simulink model "Follow_Gap_Computation_2023a"  (R2023a)
settings: Solver=ode3  StartTime=0.0  StopTime=inf  FixedStep=0.05  RelTol=1e-3
libraries: robotlib x4
settings Model: Creator=pmodi  LastModifiedBy=gptp
settings OptimizationCC: EnhancedBackFolding=on  PassReuseOutputArgsAs=Individual arguments  ZeroExternalMemoryAtStartup=off  ZeroInternalMemoryAtStartup=off  MaxStackSize=64  OptimizeBlockOrder=speed  DifferentSizesBufferReuse=on  OptimizationCustomize=off  EfficientTunableParamExpr=on
settings DebuggingCC: ParameterTunabilityLossMsg=error
settings HardwareCC: ProdBitPerLong=64  ProdLargestAtomicInteger=LongLong  ProdLargestAtomicFloat=Double  ProdLongLongMode=on  ProdHWDeviceType=ARM Compatible->ARM 64-bit (LP64)
settings SFSimCC: MATLABDynamicMemAlloc=off
settings RTWCC: Description=Embedded Coder  SystemTargetFile=ert.tlc  HardwareBoard=Robot Operating System (ROS)  TLCOptions="-aInlineSetEventsForThisBaseRateFcn=TLC_FALSE -aSuppressMultiTaskScheduler=TLC_FALSE  -aRateBasedStepFcn=0"  GenCodeOnly=on  TemplateMakefile=ert_default_tmf  Toolchain=Catkin  TargetLang=C++
settings CodeAppCC: ForceParamTrailComments=on  IgnoreCustomStorageClasses=off  OperatorAnnotations=on  SimulinkDataObjDesc=on  SFDataObjDesc=on  InsertBlockDesc=on
settings ERTTargetCC: SupportVariableSizeSignals=on

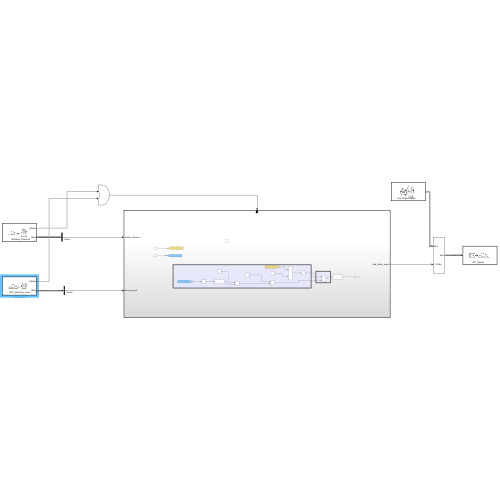
[thumbnail: Simulink's stored preview of the top-level diagram]
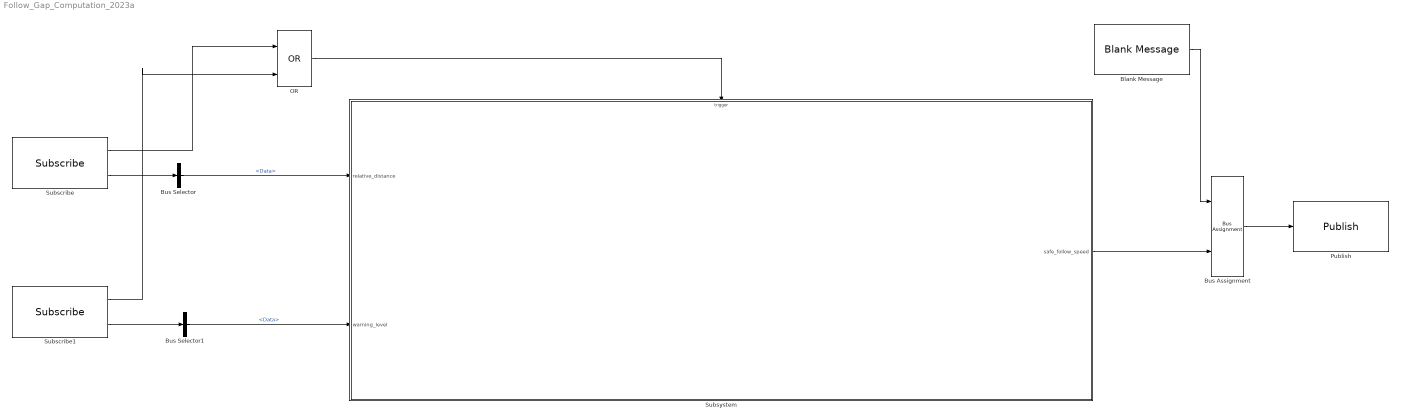
== system Follow_Gap_Computation_2023a ==
  Blank Message : robotlib/Blank Message  messageClass=Message  entityType=std_msgs/Float32  messageType=std_msgs/Float32  SampleTime=inf  legacyBusStruct=off
  Bus Assignment : BusAssignment  AssignedSignals=Data
  Bus Selector : BusSelector  OutputSignals=Data
  Bus Selector1 : BusSelector  OutputSignals=Data
  OR : Logic  Operator=OR  IconShape=distinctive  AllPortsSameDT=off  OutDataTypeStr=boolean
  Publish : robotlib/Publish  topicSource=Specify your own  topic=/SF_Speed  messageType=std_msgs/Float32  legacyBusStruct=off  messageQueueLength=1
  Subscribe : robotlib/Subscribe  topicSource=Specify your own  topic=/Relative_Distance  messageType=std_msgs/Float32  SampleTime=-1  legacyBusStruct=off  messageQueueLength=1
  Subscribe1 : robotlib/Subscribe  topicSource=Specify your own  topic=/V2V_Warning_Level  messageType=std_msgs/UInt8  SampleTime=-1  legacyBusStruct=off  messageQueueLength=1
  Subsystem : Subsystem
  wires:
  Subscribe/2 -> Bus Selector/1
  Bus Selector/1 -> Subsystem/1(relative_distance)  "<Data>"
  Bus Selector1/1 -> Subsystem/2(warning_level)  "<Data>"
  Subscribe1/2 -> Bus Selector1/1
  Blank Message/1 -> Bus Assignment/1
  Subsystem/1(safe_follow_speed) -> Bus Assignment/2
  Bus Assignment/1 -> Publish/1
  Subscribe/1 -> OR/1
  Subscribe1/1 -> OR/2
  OR/1 -> Subsystem/Trigger

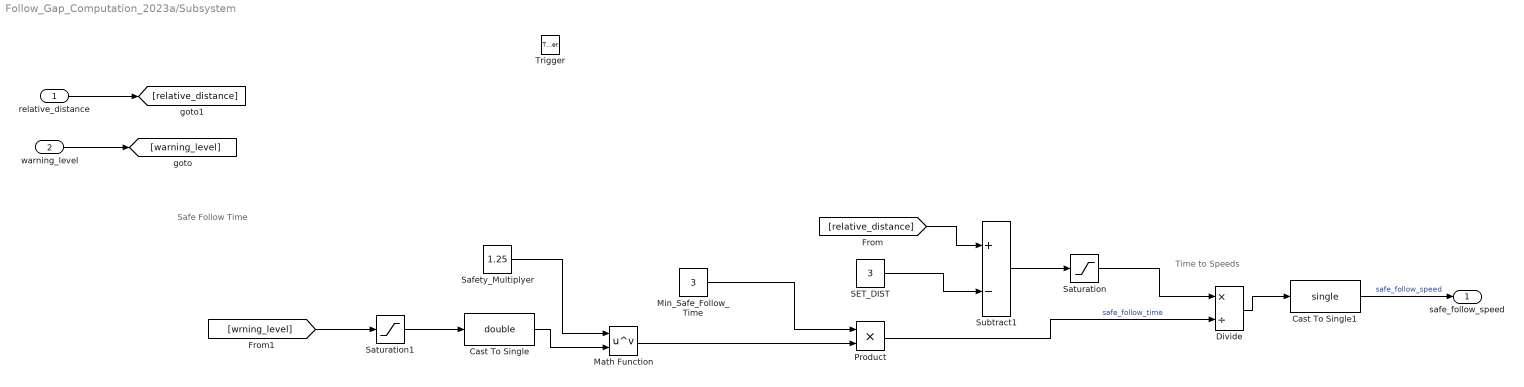
== system Follow_Gap_Computation_2023a/Subsystem ==
  note: Time to Speeds
  note: Safe Follow Time
  relative_distance : Inport
  warning_level : Inport  Port=2  OutDataTypeStr=uint8
  Trigger : TriggerPort  VariantControl=(inherit)  PortDimensions=1
  Cast To Single : DataTypeConversion  OutDataTypeStr=double  SaturateOnIntegerOverflow=off  RndMeth=Floor
  Cast To Single1 : DataTypeConversion  OutDataTypeStr=single  SaturateOnIntegerOverflow=off  RndMeth=Floor
  Divide : Product  Inputs=*/
  Math Function : Math  Operator=pow
  Min_Safe_Follow_Time : Constant  Value=3
  Product : Product
  SET_DIST : Constant  Value=3
  Safety_Multiplyer : Constant  Value=1.25
  Saturation : Saturate  UpperLimit=inf  LowerLimit=0
  Saturation1 : Saturate  UpperLimit=10  LowerLimit=0
  Subtract1 : Sum  Inputs=+-
  safe_follow_speed : Outport  OutDataTypeStr=single
  wires:
  Subtract1/1 -> Saturation/1
  Divide/1 -> Cast To Single1/1
  [relative_distance] -> Subtract1/1
  Math Function/1 -> Product/2
  Saturation/1 -> Divide/1
  relative_distance/1 -> [relative_distance]
  SET_DIST/1 -> Subtract1/2
  warning_level/1 -> [warning_level]
  Safety_Multiplyer/1 -> Math Function/1
  Min_Safe_Follow_Time/1 -> Product/1
  Cast To Single/1 -> Math Function/2
  [wrning_level] -> Saturation1/1
  Saturation1/1 -> Cast To Single/1
  Product/1 -> Divide/2  "safe_follow_time"
  Cast To Single1/1 -> safe_follow_speed/1  "safe_follow_speed"
